simulink library "filteredPIDController"  (R2020a)
settings: Solver=VariableStepAuto  StartTime=0.0  StopTime=10.0  RelTol=1e-3
values from neighbouring files (symbols this model uses):
  tau = 0.381966    [BFGS.m]
undefined symbols (not defined in the file or in its folder): kd, ki, kp
settings Model: Creator=mcobb  LastModifiedBy=Ayaz
settings DataIOCC: ReturnWorkspaceOutputs=off
settings DebuggingCC: ArithmeticOperatorsInVariantConditions=warning
settings SFSimCC: CustomCodeUndefinedFunction=UseInterfaceOnly

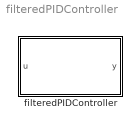
== system filteredPIDController ==
  filteredPIDController : Subsystem  mask{kp=kp, ki=ki, kd=kd, Value=tau, externalReset=none}
      mask prompts: kp "Proportional Gain, kp"; ki "Integral Gain, ki"; kd "Derivative Gain, kd"; Value "Time Constant, s"; externalReset "External reset:"
      mask init:
      | i0=find_system(gcb,'LookUnderMasks','on','FollowLinks','on','Name','Integrator');
      | i0=getSimulinkBlockHandle(i0{1});
      | i1=find_system(gcb,'LookUnderMasks','on','FollowLinks','on','Name','Integrator1');
      | i1=getSimulinkBlockHandle(i1{1});
      | i2=find_system(gcb,'LookUnderMasks','on','FollowLinks','on','Name','Integrator2');
      | i2=getSimulinkBlockHandle(i2{1});
      | rst=find_system(gcb,'LookUnderMasks','on','FollowLinks','on','Name','rst');
      | if ~isempty(rst)
      |     rst=getSimulinkBlockHandle(rst{1});
      | end
      | set_param(i0,'externalReset',externalReset)
      | set_param(i1,'externalReset',externalReset)
      | set_param(i2,'externalReset',externalReset)
      | if externalReset == "none" && ~isempty(rst)
      |     h=get_param([gcb,'/rst'],'lineHandles');
      |     delete_line(h.Outport(1));
      |     delete_block([gcb,'/rst']);
      | elseif externalReset ~= "none" && isempty(rst)
      |     add_block('built-in/Inport',[gcb,'/rst']);
      |     set_param([gcb,'/rst'],'position',[75   255   125   305])
      |     add_line(gcb,'rst/1',[get_param(i0,'Name'),'/2'])
      |     add_line(gcb,'rst/1',[get_param(i1,'Name'),'/2'])
      |     add_line(gcb,'rst/1',[get_param(i2,'Name'),'/2'])
      | end
      mask TypeOptions kp: kp/Gain
      mask TypeOptions ki: ki/Gain
      mask TypeOptions kd: kd/Gain
      mask TypeOptions Value: tau/Value
      mask TypeOptions externalReset: none | rising | falling | either | level | level hold

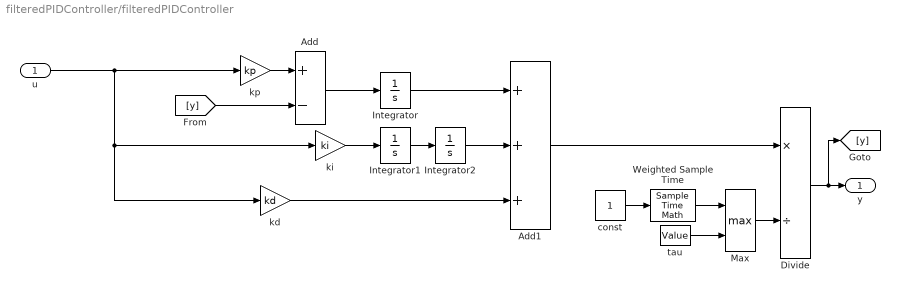
== system filteredPIDController/filteredPIDController ==
  u : Inport  PortDimensions=1
  Add : Sum  Inputs=+-
  Add1 : Sum  Inputs=+++
  Divide : Product  Inputs=*/
  Integrator : Integrator
  Integrator1 : Integrator
  Integrator2 : Integrator
  Max : MinMax  Function=max  Inputs=2
  Weighted Sample Time : SampleTimeMath  TsampMathOp=Ts Only
  const : Constant
  kd : Gain  Gain=kd
  ki : Gain  Gain=ki
  kp : Gain  Gain=kp
  tau : Constant  Value=Value
  y : Outport  PortDimensions=1  VectorParamsAs1DForOutWhenUnconnected=off
  wires:
  kp/1 -> Add/1
  [y] -> Add/2
  Add/1 -> Integrator/1
  Max/1 -> Divide/2
  tau/1 -> Max/2
  Integrator1/1 -> Integrator2/1
  ki/1 -> Integrator1/1
  u/1 -> kd/1, ki/1, kp/1
  Integrator2/1 -> Add1/2
  Integrator/1 -> Add1/1
  kd/1 -> Add1/3
  Add1/1 -> Divide/1
  Divide/1 -> [y], y/1
  Weighted Sample Time/1 -> Max/1
  const/1 -> Weighted Sample Time/1
